simulink model "questao2_prova3"  (Simulink 7.9)
settings: Solver=ode45  StartTime=0.0  StopTime=20.0  RelTol=1e-3
settings Model: Creator=Danilo  LastModifiedBy=Danilo

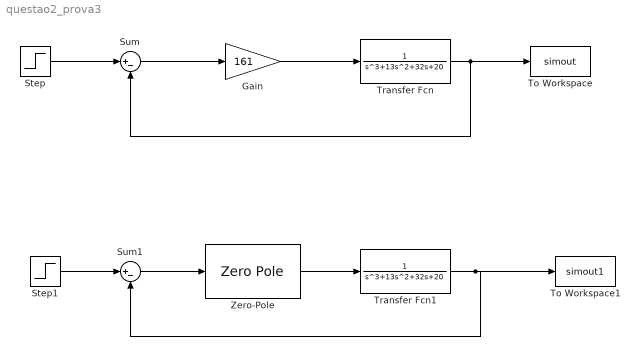
== system questao2_prova3 ==
  Gain : Gain  Gain=161
  Step : Step  Time=0  SampleTime=0
  Step1 : Step  Time=0  SampleTime=0
  Sum : Sum  Inputs=|+-
  Sum1 : Sum  Inputs=|+-
  To Workspace : ToWorkspace  VariableName=simout  SampleTime=-1
  To Workspace1 : ToWorkspace  VariableName=simout1  SampleTime=-1
  Transfer Fcn : TransferFcn  Denominator=[1 13 32 20]
  Transfer Fcn1 : TransferFcn  Denominator=[1 13 32 20]
  Zero-Pole : ZeroPole  Zeros=[-0.5584]  Poles=[-0.05]  Gain=[192]
  wires:
  Step/1 -> Sum/1
  Sum/1 -> Gain/1
  Gain/1 -> Transfer Fcn/1
  Transfer Fcn/1 -> To Workspace/1, Sum/2
  Step1/1 -> Sum1/1
  Sum1/1 -> Zero-Pole/1
  Zero-Pole/1 -> Transfer Fcn1/1
  Transfer Fcn1/1 -> To Workspace1/1, Sum1/2
